simulink model "closed_loopnew"  (R2022b)
settings: Solver=VariableStepAuto  StartTime=0.0  StopTime=10.0  RelTol=1e-3
libraries: spsControlledVoltageSourceLib x1, spsDCMachineLib x1, spsDCVoltageSourceLib x1, sps_lib x1
settings Model: Creator=happy  LastModifiedBy=Mani

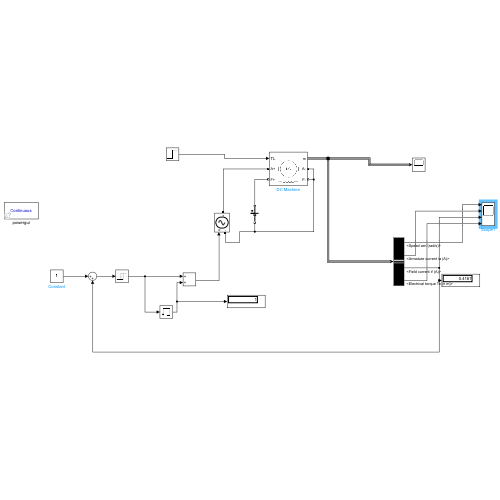
[thumbnail: Simulink's stored preview of the top-level diagram]
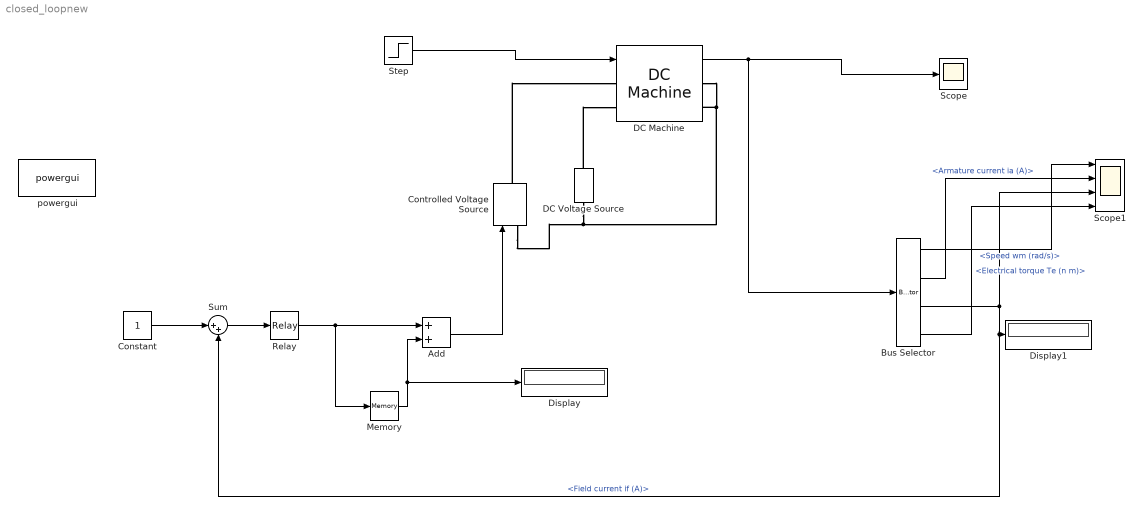
== system closed_loopnew ==
  Add : Sum
  Bus Selector : BusSelector  OutputSignals=Speed wm (rad/s),Armature current ia (A),Field current if (A),Electrical torque Te (n m)
  Constant : Constant
  Controlled Voltage Source : spsControlledVoltageSourceLib/Controlled Voltage Source  Initialize=on  Source_Type=AC  Amplitude=0  Phase=0  Frequency=0  Measurements=None
  DC Machine : spsDCMachineLib/DC Machine  PresetModel=No  MechanicalLoad=Torque TL  FieldType=Wound  ShowDetailedParameters=on  MeasurementBus=off  RLa="[ 0.6  0.012]"  RLf="[ 240  120]"  Laf=1.8  MachineConstant=Torque constant (N.m/A)  Ke=1.8  Kt=1.8  J=1  Bm=0  Tf=0  w0=1  Ifinit=0.416666666666667  TsPowergui=0  TsBlock=-1
  DC Voltage Source : spsDCVoltageSourceLib/DC Voltage Source  Amplitude=100  Measurements=None
  Display : Display
  Display1 : Display
  Memory : Memory
  Relay : Relay
  Scope : Scope
  Scope1 : Scope  NumInputPorts=4
  Step : Step  SampleTime=0
  Sum : Sum  Inputs=|++
  powergui : sps_lib/powergui  Priority=1  SimulationMode=Continuous  SampleTime=50e-6  frequency=60  Iterations=50  frequencyindice=0  Pbase=100e6  ErrMax=1e-4  UnitsV=kV  UnitsW=MW  buscounter=0  FunctionMessages=off  echomessages=off  EnableUseOfTLC=off  CurrentSourceSwitches=off  DisableSnubberDevices=off  DisableRonSwitches=off  DisableVfSwitches=off  DisplayEquations=off  AutomaticDiscreteSolvers=off  SolverType=Tustin/Backward Euler (TBE)  Interpol=off  ExternalGateDelay=off  methode=off  Ts=100  x0status=blocks  SPID=on  SwTol=0  HookPort=off  NonlinearTolerance=1e-4  nMaxIteration=100  ContinueOnMaxIteration=off  RestoreLinks=warning  ResistiveCurrentMeasurement=off  Frange=[0:2:500]  Ylog=off  Xlog=on  ShowGrid=off  save=off  variable=ZData  structure=0  ZoomFFT=off  StartTime=0.0  cycles=1  DisplayStyle=1  fundamental=60  FreqAxis=off  MaxFrequency=1000  frequencyindicesteady=1  RmsSteady=1  display=off
  wires:
  Constant/1 -> Sum/1
  Sum/1 -> Relay/1
  Relay/1 -> Memory/1, Add/1
  Memory/1 -> Add/2, Display/1
  Add/1 -> Controlled Voltage Source/1
  Step/1 -> DC Machine/1
  Bus Selector/1 -> Scope1/1  "<Speed wm (rad/s)>"
  Bus Selector/3 -> Scope1/3, Sum/2, Display1/1  "<Field current if (A)>"
  Bus Selector/4 -> Scope1/4  "<Electrical torque Te (n m)>"
  DC Machine/1 -> Bus Selector/1, Scope/1
  Bus Selector/2 -> Scope1/2  "<Armature current ia (A)>"
  connections:
  DC Voltage Source/RConn1 -- DC Machine/LConn2
  DC Machine/RConn1 -- Controlled Voltage Source/LConn1 -- DC Voltage Source/LConn1 -- DC Machine/RConn2
  Controlled Voltage Source/RConn1 -- DC Machine/LConn1
